simulink model "validacion_subsistema_mecanico"  (R2023b)
settings: Solver=VariableStepAuto  StartTime=0.0  StopTime=10.0  RelTol=1e-3
values from neighbouring files (symbols this model uses):
  beq_nom = bm + bl_nom/r^2    (= 2.19444444444e-05)    [parametros_planta.m]    (also in params_subsistema_mecanico.m; sistema_completo_en_codigo.m)
  Jeq_nom = Jm + Jl_nom/r^2    (= 1.97847222222e-05)    [params_subsistema_mecanico.m]    (also in sistema_completo_en_codigo.m)
  kg_eq_nom = g*kl_nom/r    (= 0.0204305208333)    [params_subsistema_mecanico.m]    (also in sistema_completo_en_codigo.m)
  r = 120.0    (= 120)    [controlador_foc_simulink.m]    (also in parametros_planta.m; params_subsistema_mecanico.m; sistema_completo_en_codigo.m)
settings Model: Creator=Gabriel  LastModifiedBy=Pc

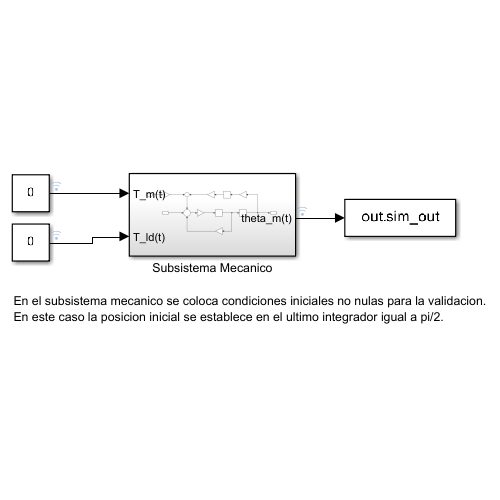
[thumbnail: Simulink's stored preview of the top-level diagram]
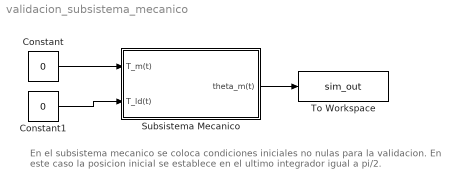
== system validacion_subsistema_mecanico ==
  note: En el subsistema mecanico se coloca condiciones iniciales no nulas para la validacion.
      | En este caso la posicion inicial se establece en el ultimo integrador igual a pi/2.
  Constant : Constant  Value=0
  Constant1 : Constant  Value=0
  Subsistema Mecanico : Subsystem
  To Workspace : ToWorkspace  VariableName=sim_out  SaveFormat=Structure With Time  SampleTime=-1
  wires:
  Subsistema Mecanico/1(theta_m(t)) -> To Workspace/1
  Constant/1 -> Subsistema Mecanico/1(T_m(t))
  Constant1/1 -> Subsistema Mecanico/2(T_ld(t))

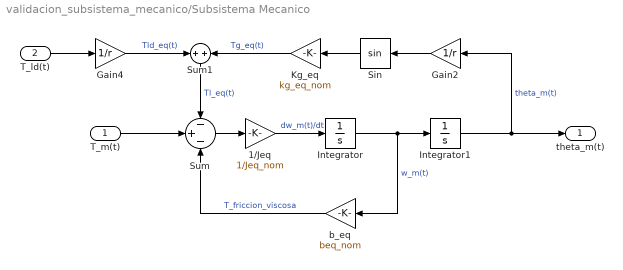
== system validacion_subsistema_mecanico/Subsistema Mecanico ==
  T_m(t) : Inport
  T_ld(t) : Inport  Port=2
  1/Jeq : Gain  Gain=1/Jeq_nom
  Gain2 : Gain  Gain=1/r
  Gain4 : Gain  Gain=1/r
  Integrator : Integrator
  Integrator1 : Integrator  InitialCondition=pi/2
  Kg_eq : Gain  Gain=kg_eq_nom
  Sin : Trigonometry
  Sum : Sum  Inputs=-+-
  Sum1 : Sum  Inputs=+|+
  b_eq : Gain  Gain=beq_nom
  theta_m(t) : Outport
  wires:
  Gain2/1 -> Sin/1
  Sum1/1 -> Sum/1  "Tl_eq(t)"
  Gain4/1 -> Sum1/1  "Tld_eq(t)"
  Integrator1/1 -> theta_m(t)/1, Gain2/1  "theta_m(t)"
  T_m(t)/1 -> Sum/2
  Kg_eq/1 -> Sum1/2  "Tg_eq(t)"
  b_eq/1 -> Sum/3  "T_friccion_viscosa"
  T_ld(t)/1 -> Gain4/1
  Sin/1 -> Kg_eq/1
  Sum/1 -> 1/Jeq/1
  Integrator/1 -> b_eq/1, Integrator1/1  "w_m(t)"
  1/Jeq/1 -> Integrator/1  "dw_m(t)/dt"
